simulink model "HW5_sim"  (R2022b)
settings: Solver=VariableStepAuto  StartTime=0.0  StopTime=10.0  RelTol=1e-3
undefined symbols (not defined in the file): b_p, b_theta, b_z, f_theta, f_z, J_p, K_is_theta, K_isz, K_s_theta, K_sz, K_t, K_theta, L, theta_mag, z_mag
settings Model: Creator=qingchuanhou  LastModifiedBy=qingchuanhou

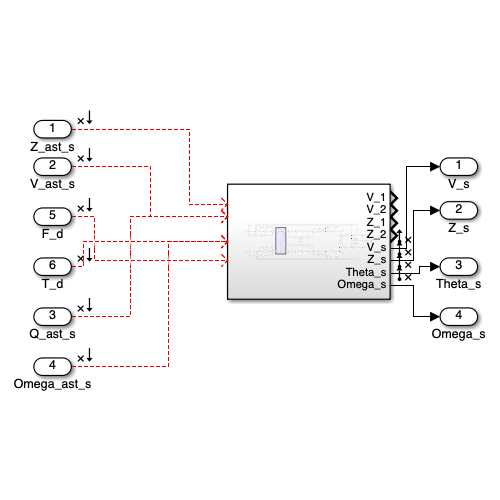
[thumbnail: Simulink's stored preview of the top-level diagram]
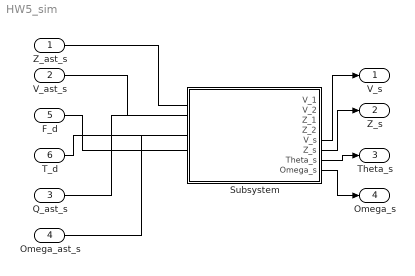
== system HW5_sim ==
  Z_ast_s : Inport
  V_ast_s : Inport  Port=2
  Q_ast_s : Inport  Port=3
  Omega_ast_s : Inport  Port=4
  F_d : Inport  Port=5
  T_d : Inport  Port=6
  Subsystem : Subsystem
  V_s : Outport
  Z_s : Outport  Port=2
  Theta_s : Outport  Port=3
  Omega_s : Outport  Port=4
  wires:
  Omega_ast_s/1 -> ?
  Subsystem/6(Z_s) -> Z_s/1
  V_ast_s/1 -> ?
  F_d/1 -> ?
  Subsystem/7(Theta_s) -> Theta_s/1
  Subsystem/5(V_s) -> V_s/1
  Z_ast_s/1 -> ?
  Q_ast_s/1 -> ?
  Subsystem/8(Omega_s) -> Omega_s/1
  T_d/1 -> ?

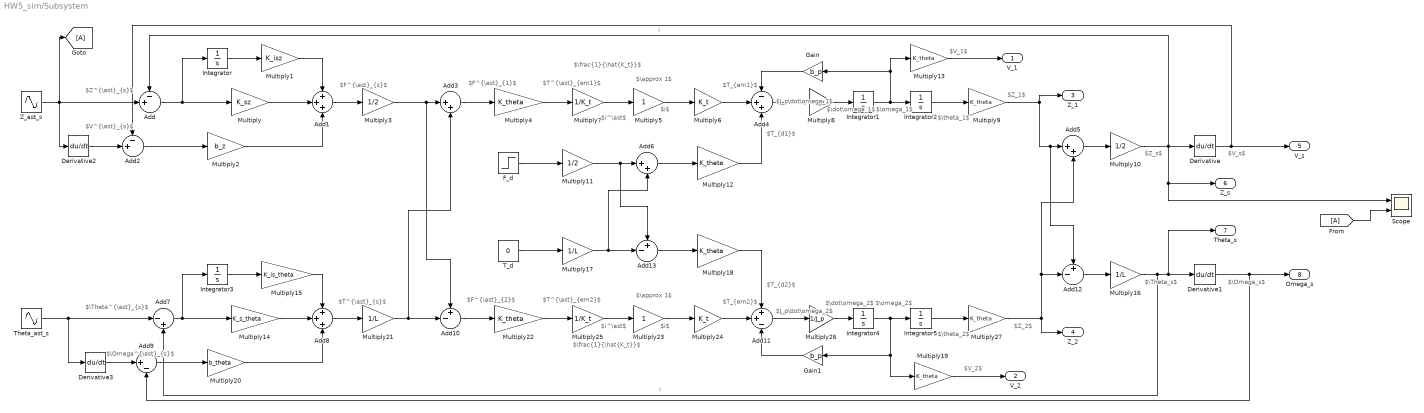
== system HW5_sim/Subsystem ==
  note: $\approx 1$
  note: $\frac{1}{\hat{K_t}}$
  note: $\omega_1$
  note: $Z_s$
  note: $V_s$
  note: $Z_1$
  note: $\theta_1$
  note: $\dot\omega_1$
  note: $V_1$
  note: $i^\ast$
  note: $i$
  note: $T_{em1}$
  note: $T^{\ast}_{em1}$
  note: $F^{\ast}_{s}$
  note: $F^{\ast}_{1}$
  note: $Z^{\ast}_{s}$
  note: $V^{\ast}_{s}$
  note: $\frac{1}{\hat{K_t}}$
  note: $\Omega_s$
  note: $V_2$
  note: $T^{\ast}_{em2}$
  note: $\Theta_s$
  note: $\omega_2$
  note: $\dot\omega_2$
  note: $i$
  note: $i^\ast$
  note: $\approx 1$
  note: $T^{\ast}_{s}$
  note: $T_{em2}$
  note: $\theta_2$
  note: $Z_2$
  note: $F^{\ast}_{2}$
  note: $\Theta^{\ast}_{s}$
  note: $\Omega^{\ast}_{s}$
  note: $J_p\dot\omega_2$
  note: $J_p\dot\omega_1$
  note: $T_{d2}$
  note: $T_{d1}$
  Add : Sum  Inputs=-+|
  Add1 : Sum  Inputs=+++
  Add10 : Sum  Inputs=+-|
  Add11 : Sum  Inputs=++-
  Add12 : Sum  Inputs=+-|
  Add13 : Sum  Inputs=+-|
  Add2 : Sum  Inputs=-+|
  Add3 : Sum  Inputs=|++
  Add4 : Sum  Inputs=-++
  Add5 : Sum  Inputs=|++
  Add6 : Sum  Inputs=|++
  Add7 : Sum  Inputs=|-+
  Add8 : Sum  Inputs=+++
  Add9 : Sum  Inputs=|+-
  Derivative{,1..3} (4 alike) : Derivative
  F_d : Step  After=1000  SampleTime=0
  From : From
  Gain : Gain  Gain=b_p
  Gain1 : Gain  Gain=b_p
  Goto : Goto
  Integrator{,1..5} (6 alike) : Integrator
  Multiply : Gain  Gain=K_sz
  Multiply1 : Gain  Gain=K_isz
  Multiply10 : Gain  Gain=1/2
  Multiply11 : Gain  Gain=1/2
  Multiply{4,9,12..13,18..19,22,27} (8 alike) : Gain  Gain=K_theta
  Multiply14 : Gain  Gain=K_s_theta
  Multiply15 : Gain  Gain=K_is_theta
  Multiply16 : Gain  Gain=1/L
  Multiply17 : Gain  Gain=1/L
  Multiply2 : Gain  Gain=b_z
  Multiply20 : Gain  Gain=b_theta
  Multiply21 : Gain  Gain=1/L
  Multiply23 : Gain
  Multiply24 : Gain  Gain=K_t
  Multiply25 : Gain  Gain=1/K_t
  Multiply26 : Gain  Gain=1/J_p
  Multiply3 : Gain  Gain=1/2
  Multiply5 : Gain
  Multiply6 : Gain  Gain=K_t
  Multiply7 : Gain  Gain=1/K_t
  Multiply8 : Gain  Gain=1/J_p
  Scope : Scope  NumInputPorts=2
  T_d : Constant  Value=0
  Theta_ast_s : Sin  Amplitude=theta_mag  Frequency=2*pi*f_theta  SampleTime=0
  Z_ast_s : Sin  Amplitude=z_mag  Frequency=2*pi*f_z  SampleTime=0
  V_1 : Outport
  V_2 : Outport  Port=2
  Z_1 : Outport  Port=3
  Z_2 : Outport  Port=4
  V_s : Outport  Port=5
  Z_s : Outport  Port=6
  Theta_s : Outport  Port=7
  Omega_s : Outport  Port=8
  wires:
  Multiply19/1 -> V_2/1
  Add9/1 -> Multiply20/1
  Add12/1 -> Multiply16/1
  Multiply23/1 -> Multiply24/1
  Add5/1 -> Multiply10/1
  Integrator2/1 -> Multiply9/1
  Multiply20/1 -> Add8/3
  Integrator5/1 -> Multiply27/1
  Integrator/1 -> Multiply1/1
  Z_ast_s/1 -> Goto/1, Derivative2/1, Add/2
  Gain/1 -> Add4/1
  Gain1/1 -> Add11/3
  Multiply24/1 -> Add11/2
  Integrator3/1 -> Multiply15/1
  Add10/1 -> Multiply22/1
  Multiply14/1 -> Add8/2
  Multiply7/1 -> Multiply5/1
  Multiply15/1 -> Add8/1
  Add13/1 -> Multiply18/1
  Multiply1/1 -> Add1/1
  Integrator1/1 -> Gain/1, Multiply13/1, Integrator2/1
  Multiply8/1 -> Integrator1/1
  Multiply22/1 -> Multiply25/1
  Theta_ast_s/1 -> Add7/1, Derivative3/1
  Multiply3/1 -> Add3/1, Add10/1
  Add7/1 -> Integrator3/1, Multiply14/1
  Multiply26/1 -> Integrator4/1
  T_d/1 -> Multiply17/1
  Multiply25/1 -> Multiply23/1
  Derivative/1 -> V_s/1, Add2/1
  F_d/1 -> Multiply11/1
  Multiply21/1 -> Add10/2, Add3/2
  Integrator4/1 -> Multiply19/1, Gain1/1, Integrator5/1
  Multiply9/1 -> Z_1/1, Add5/1, Add12/1
  Multiply2/1 -> Add1/3
  Derivative1/1 -> Omega_s/1, Add9/2
  Multiply13/1 -> V_1/1
  Multiply5/1 -> Multiply6/1
  Multiply10/1 -> Derivative/1, Scope/1, Z_s/1, Add/1  "i"
  Add4/1 -> Multiply8/1
  Multiply/1 -> Add1/2
  Multiply6/1 -> Add4/2
  Multiply12/1 -> Add4/3
  Add2/1 -> Multiply2/1
  Multiply27/1 -> Z_2/1, Add12/2, Add5/2
  Add1/1 -> Multiply3/1
  Multiply16/1 -> Theta_s/1, Derivative1/1, Add7/2  "i"
  Multiply4/1 -> Multiply7/1
  Add3/1 -> Multiply4/1
  Add8/1 -> Multiply21/1
  Add6/1 -> Multiply12/1
  Add11/1 -> Multiply26/1
  Multiply11/1 -> Add6/1, Add13/1
  Multiply18/1 -> Add11/1
  Add/1 -> Integrator/1, Multiply/1
  Multiply17/1 -> Add6/2, Add13/2
  Derivative2/1 -> Add2/2
  Derivative3/1 -> Add9/1
  From/1 -> Scope/2
